simulink model "Wind_DC_Battery_Complete"  (R2022a)
settings: Solver=daessc  StartTime=0.0  StopTime=3600*24  MaxStep=60/10  RelTol=1e-3  AbsTol=1e-3
undefined symbols (not defined in the file or in its folder): Battery, Electric, Generator, Plate, R_h2, Setpoint
libraries: fl_lib x63, nesl_utility x18, ee_lib x5, simulink x1, sdl_lib x1
(part 2 of 5)

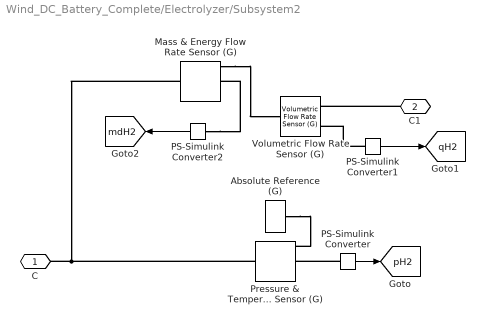
== system Wind_DC_Battery_Complete/Electrolyzer/Subsystem2 ==
  Absolute Reference (G) : fl_lib/Gas/Elements/Absolute Reference (G)
      settings: SourceProductBaseCode=PW,SS,VE  InternalSimscapePortConfiguration="{\"Bottom\":[],\"Left\":[{\"id\":\"A\",\"label\":\"\",\"type\":\"foundation.gas.gas\"}],\"Right\":[],\"Top\":[]}"
  Mass & Energy Flow Rate Sensor (G) : fl_lib/Gas/Sensors/Mass & Energy Flow Rate Sensor (G)
      settings: SourceProductBaseCode=PW,SS,VE  InternalSimscapePortConfiguration="{\"Bottom\":[],\"Left\":[{\"id\":\"A\",\"label\":\"A\",\"type\":\"foundation.gas.gas\"}],\"Right\":[{\"id\":\"B\",\"label\":\"B\",\"type\":\"foundation.gas.gas\"},{\"id\":\"M\",\"label\":\"M\",\"type\":\"output\"},{\"id\":\"PHI\",\"label\":\"Phi\",\"type\":\"output\"}],\"Top\":[]}"
  PS-Simulink Converter : nesl_utility/PS-Simulink Converter  PhysicalDomain=network_engine_domain  SubClassName=ps_output  LeftPortType=input  RightPortType=output  PseudoPeriodic=off  Frequencies=[]  VectorFormat=1-D array  Unit=bar  AffineConversion=off
      settings: SourceProductBaseCode=SS,PW,VE
  PS-Simulink Converter1 : nesl_utility/PS-Simulink Converter  PhysicalDomain=network_engine_domain  SubClassName=ps_output  LeftPortType=input  RightPortType=output  PseudoPeriodic=off  Frequencies=[]  VectorFormat=1-D array  Unit=m^3/hr  AffineConversion=off
      settings: SourceProductBaseCode=SS,PW,VE
  PS-Simulink Converter2 : nesl_utility/PS-Simulink Converter  PhysicalDomain=network_engine_domain  SubClassName=ps_output  LeftPortType=input  RightPortType=output  PseudoPeriodic=off  Frequencies=[]  VectorFormat=1-D array  Unit=kg/hr  AffineConversion=off
      settings: SourceProductBaseCode=SS,PW,VE
  Pressure & Temperature Sensor (G) : fl_lib/Gas/Sensors/Pressure & Temperature Sensor (G)
      settings: SourceProductBaseCode=PW,SS,VE  InternalSimscapePortConfiguration="{\"Bottom\":[],\"Left\":[{\"id\":\"A\",\"label\":\"A\",\"type\":\"foundation.gas.gas\"}],\"Right\":[{\"id\":\"B\",\"label\":\"B\",\"type\":\"foundation.gas.gas\"},{\"id\":\"P\",\"label\":\"P\",\"type\":\"output\"},{\"id\":\"T\",\"label\":\"T\",\"type\":\"output\"}],\"Top\":[]}"
  Volumetric Flow Rate Sensor (G) : fl_lib/Gas/Sensors/Volumetric Flow Rate Sensor (G)
      settings: SourceProductBaseCode=PW,SS,VE  InternalSimscapePortConfiguration="{\"Bottom\":[],\"Left\":[{\"id\":\"A\",\"label\":\"A\",\"type\":\"foundation.gas.gas\"}],\"Right\":[{\"id\":\"B\",\"label\":\"B\",\"type\":\"foundation.gas.gas\"},{\"id\":\"V\",\"label\":\"V\",\"type\":\"output\"}],\"Top\":[]}"
  C : PMIOPort  Side=Left
  C1 : PMIOPort  Port=2  Side=Left
  tag scope: mdH2=global, pH2=global, qH2=global
  wires:
  PS-Simulink Converter/1 -> [pH2]
  PS-Simulink Converter1/1 -> [qH2]
  PS-Simulink Converter2/1 -> [mdH2]
  connections:
  PS-Simulink Converter/LConn1 -- Pressure & Temperature Sensor (G)/RConn2
  Pressure & Temperature Sensor (G)/LConn1 -- Mass & Energy Flow Rate Sensor (G)/LConn1 -- C/RConn1
  Absolute Reference (G)/LConn1 -- Pressure & Temperature Sensor (G)/RConn1
  C1/RConn1 -- Volumetric Flow Rate Sensor (G)/RConn1
  PS-Simulink Converter1/LConn1 -- Volumetric Flow Rate Sensor (G)/RConn2
  Mass & Energy Flow Rate Sensor (G)/RConn1 -- Volumetric Flow Rate Sensor (G)/LConn1
  PS-Simulink Converter2/LConn1 -- Mass & Energy Flow Rate Sensor (G)/RConn2

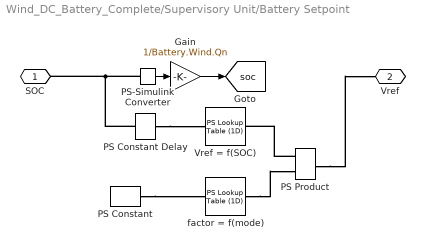
== system Wind_DC_Battery_Complete/Supervisory Unit/Battery Setpoint ==
  Gain : Gain  Gain=1/Battery.Wind.Qn
  PS Constant : fl_lib/Physical Signals/Sources/PS Constant  constant=bat_mode
      settings: SourceProductBaseCode=PW,SS,VE
  PS Constant Delay : fl_lib/Physical Signals/Delays/PS Constant Delay  InputHistory=Battery.Wind.Qn A*hr  DelayTime=60 s
      settings: SourceProductBaseCode=PW,SS,VE  InternalSimscapePortConfiguration="{\"Bottom\":[],\"Left\":[{\"id\":\"U\",\"label\":\"U\",\"type\":\"input\"}],\"Right\":[{\"id\":\"Y\",\"label\":\"Y\",\"type\":\"output\"}],\"Top\":[]}"
  PS Product : fl_lib/Physical Signals/Functions/PS Product
      settings: SourceProductBaseCode=PW,SS,VE
  PS-Simulink Converter : nesl_utility/PS-Simulink Converter  PhysicalDomain=network_engine_domain  SubClassName=ps_output  LeftPortType=input  RightPortType=output  PseudoPeriodic=off  Frequencies=[]  VectorFormat=1-D array  Unit=A*hr  AffineConversion=off
      settings: SourceProductBaseCode=SS,PW,VE
  Vref = f(SOC) : fl_lib/Physical Signals/Lookup Tables/PS Lookup Table (1D)  x=Battery.Wind.SOC_Vect A*hr  f=Battery.Wind.Vref_Vect V  interp_method=simscape.enum.interpolation.linear  extrap_method=simscape.enum.extrapolation.linear
      settings: SourceProductBaseCode=PW,SS,VE
  factor = f(mode) : fl_lib/Physical Signals/Lookup Tables/PS Lookup Table (1D)  x=[0 1]  f=[0.8 1]  interp_method=simscape.enum.interpolation.linear  extrap_method=simscape.enum.extrapolation.nearest
      settings: SourceProductBaseCode=PW,SS,VE
  SOC : PMIOPort  Side=Left
  Vref : PMIOPort  Port=2  Side=Right
  tag scope: soc=global
  wires:
  PS-Simulink Converter/1 -> Gain/1
  Gain/1 -> [soc]
  connections:
  PS-Simulink Converter/LConn1 -- SOC/RConn1 -- PS Constant Delay/LConn1
  PS Constant Delay/RConn1 -- Vref = f(SOC)/LConn1
  PS Product/LConn1 -- Vref = f(SOC)/RConn1
  PS Product/RConn1 -- Vref/RConn1
  factor = f(mode)/RConn1 -- PS Product/LConn2
  PS Constant/RConn1 -- factor = f(mode)/LConn1

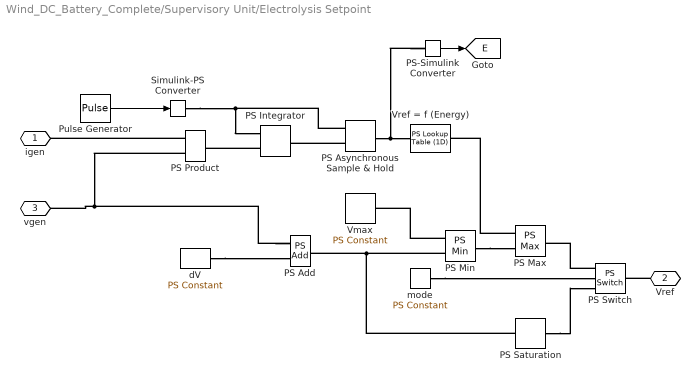
== system Wind_DC_Battery_Complete/Supervisory Unit/Electrolysis Setpoint  ==
  PS Add : fl_lib/Physical Signals/Functions/PS Add
      settings: SourceProductBaseCode=PW,SS,VE
  PS Asynchronous Sample & Hold : fl_lib/Physical Signals/Discrete/PS Asynchronous Sample & Hold  Y0=50 kW*hr
      settings: SourceProductBaseCode=PW,SS,VE  InternalSimscapePortConfiguration="{\"Bottom\":[],\"Left\":[{\"id\":\"U\",\"label\":\"\",\"type\":\"input\"},{\"id\":\"T\",\"label\":\"\",\"type\":\"input\"}],\"Right\":[{\"id\":\"Y\",\"label\":\"\",\"type\":\"output\"}],\"Top\":[]}"
  PS Integrator : fl_lib/Physical Signals/Linear Operators/PS Integrator  reset_method=foundation.enum.IntegratorResetSpec.Rising  initial_condition_spec=foundation.enum.IntegratorICSpec.Internal  x0=0 kW*hr
      settings: SourceProductBaseCode=PW,SS,VE  InternalSimscapePortConfiguration="{\"Bottom\":[],\"Left\":[{\"id\":\"I\",\"label\":\"\",\"type\":\"input\"},{\"id\":\"R\",\"label\":\"R\",\"type\":\"input\"}],\"Right\":[{\"id\":\"O\",\"label\":\"\",\"type\":\"output\"}],\"Top\":[]}"
  PS Max : fl_lib/Physical Signals/Nonlinear Operators/PS Max
      settings: SourceProductBaseCode=PW,SS,VE  InternalSimscapePortConfiguration="{\"Bottom\":[],\"Left\":[{\"id\":\"I1\",\"label\":\"\",\"type\":\"input\"},{\"id\":\"I2\",\"label\":\"\",\"type\":\"input\"}],\"Right\":[{\"id\":\"O\",\"label\":\"\",\"type\":\"output\"}],\"Top\":[]}"
  PS Min : fl_lib/Physical Signals/Nonlinear Operators/PS Min
      settings: SourceProductBaseCode=PW,SS,VE  InternalSimscapePortConfiguration="{\"Bottom\":[],\"Left\":[{\"id\":\"I1\",\"label\":\"\",\"type\":\"input\"},{\"id\":\"I2\",\"label\":\"\",\"type\":\"input\"}],\"Right\":[{\"id\":\"O\",\"label\":\"\",\"type\":\"output\"}],\"Top\":[]}"
  PS Product : fl_lib/Physical Signals/Functions/PS Product
      settings: SourceProductBaseCode=PW,SS,VE
  PS Saturation : fl_lib/Physical Signals/Nonlinear Operators/PS Saturation  upper_limit=Setpoint.Vmax V  lower_limit=Setpoint.Vmin V
      settings: SourceProductBaseCode=PW,SS,VE
  PS Switch : fl_lib/Physical Signals/Nonlinear Operators/PS Switch  Threshold=0
      settings: SourceProductBaseCode=PW,SS,VE  InternalSimscapePortConfiguration="{\"Bottom\":[],\"Left\":[{\"id\":\"I1\",\"label\":\"\",\"type\":\"input\"},{\"id\":\"I2\",\"label\":\"\",\"type\":\"input\"},{\"id\":\"I3\",\"label\":\"\",\"type\":\"input\"}],\"Right\":[{\"id\":\"O\",\"label\":\"\",\"type\":\"output\"}],\"Top\":[]}"
  PS-Simulink Converter : nesl_utility/PS-Simulink Converter  PhysicalDomain=network_engine_domain  SubClassName=ps_output  LeftPortType=input  RightPortType=output  PseudoPeriodic=off  Frequencies=[]  VectorFormat=1-D array  Unit=inherit  AffineConversion=off
      settings: SourceProductBaseCode=SS,PW,VE
  Pulse Generator : DiscretePulseGenerator  PulseType=Time based  Period=Setpoint.TimeStep  PulseWidth=50
  Simulink-PS Converter : nesl_utility/Simulink-PS Converter  PhysicalDomain=network_engine_domain  SubClassName=ps_input  LeftPortType=input  RightPortType=output  PseudoPeriodic=off  Frequencies=[]  NoiseDistribution=none  NoiseParameters=[]  Unit=1  AffineConversion=off  FilteringAndDerivatives=provide  SimscapeFilterOrder=1  InputFilterTimeConstant=0.001  UdotUserProvided=0
      settings: SourceProductBaseCode=SS,PW,VE
  Vmax : fl_lib/Physical Signals/Sources/PS Constant  constant=Setpoint.Vmax V
      settings: SourceProductBaseCode=PW,SS,VE
  Vref = f (Energy) : fl_lib/Physical Signals/Lookup Tables/PS Lookup Table (1D)  x=Setpoint.Energy_vect kW*hr  f=Setpoint.Vref_vect V  interp_method=simscape.enum.interpolation.linear  extrap_method=simscape.enum.extrapolation.nearest
      settings: SourceProductBaseCode=PW,SS,VE
  dV : fl_lib/Physical Signals/Sources/PS Constant  constant=Setpoint.dV V
      settings: SourceProductBaseCode=PW,SS,VE
  mode : fl_lib/Physical Signals/Sources/PS Constant  constant=constant
      settings: SourceProductBaseCode=PW,SS,VE
      settings: AttributesFormatString=|
      | 1: Energy
      | -1: Voltage
  igen : PMIOPort  Side=Left
  Vref : PMIOPort  Port=2  Side=Right
  vgen : PMIOPort  Port=3  Side=Left
  tag scope: E=global
  wires:
  Pulse Generator/1 -> Simulink-PS Converter/1
  PS-Simulink Converter/1 -> [E]
  connections:
  PS Add/LConn1 -- vgen/RConn1 -- PS Product/LConn2
  PS Asynchronous Sample & Hold/RConn1 -- PS-Simulink Converter/LConn1 -- Vref = f (Energy)/LConn1
  dV/RConn1 -- PS Add/LConn2
  PS Asynchronous Sample & Hold/LConn1 -- PS Integrator/RConn1
  PS Max/LConn1 -- Vref = f (Energy)/RConn1
  PS Min/RConn1 -- PS Max/LConn2
  Simulink-PS Converter/RConn1 -- PS Integrator/LConn2 -- PS Asynchronous Sample & Hold/LConn2
  PS Integrator/LConn1 -- PS Product/RConn1
  PS Min/LConn1 -- Vmax/RConn1
  PS Min/LConn2 -- PS Saturation/LConn1 -- PS Add/RConn1
  PS Product/LConn1 -- igen/RConn1
  Vref/RConn1 -- PS Switch/RConn1
  PS Switch/LConn1 -- PS Max/RConn1
  PS Saturation/RConn1 -- PS Switch/LConn3
  mode/RConn1 -- PS Switch/LConn2

== system Wind_DC_Battery_Complete/Supervisory Unit/Switch Logic ==
  Battery Recharge : fl_lib/Physical Signals/Lookup Tables/PS Lookup Table (1D)  x=[0 1 1.001 2]  f=[0 0 1 1]  interp_method=simscape.enum.interpolation.linear  extrap_method=simscape.enum.extrapolation.nearest
      settings: SourceProductBaseCode=PW,SS,VE
  Electrolyzer On : fl_lib/Physical Signals/Lookup Tables/PS Lookup Table (1D)  x=[0 0.25 0.5 1]  f=[0 0 1 1]  interp_method=simscape.enum.interpolation.linear  extrap_method=simscape.enum.extrapolation.nearest
      settings: SourceProductBaseCode=PW,SS,VE
  One : fl_lib/Physical Signals/Sources/PS Constant  constant=1
      settings: SourceProductBaseCode=PW,SS,VE
  PS Add : fl_lib/Physical Signals/Functions/PS Add
      settings: SourceProductBaseCode=PW,SS,VE
  PS Subtract : fl_lib/Physical Signals/Functions/PS Subtract
      settings: SourceProductBaseCode=PW,SS,VE
  xW : PMIOPort  Side=Right
  u : PMIOPort  Port=2  Side=Left
  xES : PMIOPort  Port=3  Side=Right
  connections:
  PS Subtract/LConn1 -- One/RConn1
  Electrolyzer On/RConn1 -- xW/RConn1 -- PS Subtract/LConn2
  Electrolyzer On/LConn1 -- Battery Recharge/LConn1 -- u/RConn1
  PS Add/LConn1 -- PS Subtract/RConn1
  PS Add/RConn1 -- xES/RConn1
  PS Add/LConn2 -- Battery Recharge/RConn1
